simulink model "kalman"  (R2026a)
settings: Solver=FixedStepAuto  StopTime=inf  FixedStep=0.01  EnableMultiTasking=on
libraries: stm32f4xxblockslib x1, stm32blockslib x1
settings Model: STM32="{\"AnalogInput\":{\"ID\":\"1\"},\"TimerCapture\":{\"ID\":\"18\"}}"  SimulationMode=external  Creator=khunb  LastModifiedBy=POND
settings OptimizationCC: MaxStackSize=512
settings HardwareCC: ProdLargestAtomicInteger=Long  ProdLargestAtomicFloat=Double  ProdHWDeviceType=ARM Compatible->ARM Cortex-M
settings SFSimCC: SimCustomHeaderCode="#include \"hc_sr04.h\""  SimUserSources=hc_sr04.c
settings RTWCC: SystemTargetFile=ert.tlc  HardwareBoard=STM32G4xx Based  TLCOptions=-aInlineSetEventsForThisBaseRateFcn=TLC_FALSE -aSuppressMultiTaskScheduler=TLC_FALSE -aRateBasedStepFcn=1  RTWUseSimCustomCode=on  CustomHeaderCode="#include \"hc_sr04.h\""  CustomSource=hc_sr04.c  Toolchain=GNU Tools for STM32  Description=Embedded Coder
settings ERTTargetCC: ExtModeTransport=3.0  ExtModeStaticAllocSize=2048.0  CodeReplacementLibrary=ARM Cortex-M

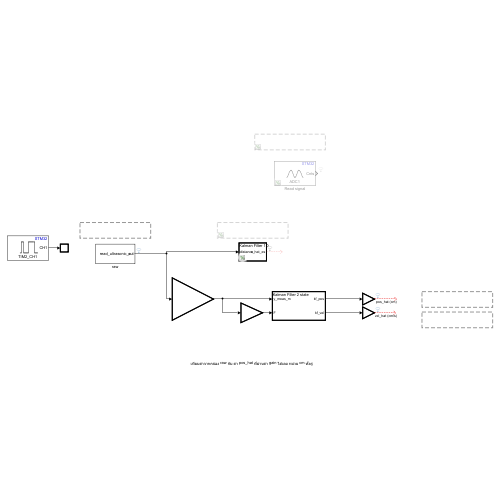
[thumbnail: Simulink's stored preview of the top-level diagram]
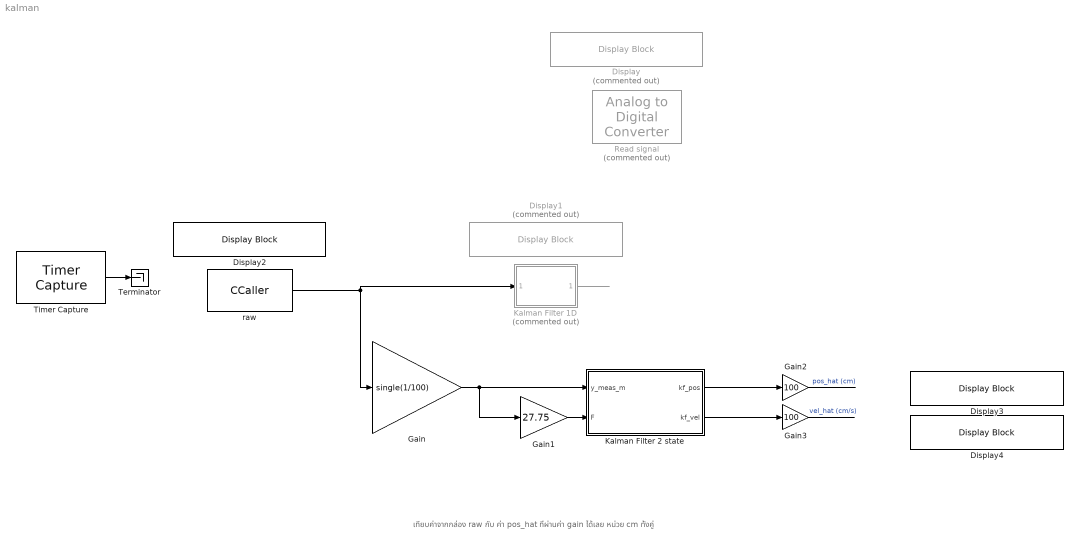
== system kalman ==
  note: เทียบค่าจากกล่อง raw กับ ค่า pos_hat ที่ผ่านค่า gain ได้เลย หน่วย cm ทั้งคู่
  Display : DisplayBlock  Commented=on  LabelPosition=Hide  Transparency=1  GridColor=[0.502, 0.502, 0.502]
  Display1 : DisplayBlock  Commented=on  LabelPosition=Hide  Transparency=1  GridColor=[0.502, 0.502, 0.502]
  Display2 : DisplayBlock  LabelPosition=Hide  Transparency=1  GridColor=[0.502, 0.502, 0.502]
  Display3 : DisplayBlock  LabelPosition=Hide  Transparency=1  GridColor=[0.502, 0.502, 0.502]
  Display4 : DisplayBlock  LabelPosition=Hide  Transparency=1  GridColor=[0.502, 0.502, 0.502]
  Gain : Gain  Gain=single(1/100)
  Gain1 : Gain  Gain=27.75
  Gain2 : Gain  Gain=100
  Gain3 : Gain  Gain=100
  Kalman Filter 1D : MATLAB Function  Commented=on  TreatAsAtomicUnit=on
  Kalman Filter 2 state : MATLAB Function  TreatAsAtomicUnit=on
  Read signal : stm32f4xxblockslib/Analog to Digital Converter  Commented=on  ADCModule=ADC1  ConversionGroup=Regular  TriggerMode=Trigger and read  NumberOfConversions=1  EnableBufferConv=off  BufferLength=1  OutputStatus=off  SampleTime=-1  EnableSimPort=off  hoistedMaskSrc=ECSoC/ECSimCodegen/Analog to Digital Converter
  Terminator : Terminator
  Timer Capture : stm32blockslib/Timer Capture  TimerModule=TIM2  SelectedChannel=CH1  CaptureLength=1  OutputDataLength=off  OutputOverrunStatus=off  OutputDirection=off  SampleTime=-1
      settings: LibrarySourceBlock=stm32g4xxblockslib/Timer Capture
  raw : CCaller  FunctionName=read_ultrasonic_c  PortSpecificationStruct="%)30     .    & (   8    (     @         %    \"     $    !     0         %  0 \"0    $    _    07)G3F%M90  4&]R=$YA;64 4V-O<&4     26YD97@     5'EP90      4VEZ90      27-';&]B86P   X    P    !@    @    $          4    (     0    ,    !         !   P!O=70 #@   #     &    \"     0         !0    @    !     P    $         $  # &]U=  .    .     8    (    !          %    \"     $    &     0         0    !@   $]U='!U=   #@   #@    &    \"     8         !0    @    !     0    $         \"0    @               X    X    !@    @    $          4    (     0    8    !         !     &    <VEN9VQE   .    ,     8    (    !          %    \"     $    !     0         0  $ ,0    X    P    !@    @    ) @        4    (     0    $    !          (  0"
  wires:
  Kalman Filter 1D/1(x_hat_es) -> ?
  raw/1 -> Kalman Filter 1D/1(distance), Gain/1
  Timer Capture/1 -> Terminator/1
  Kalman Filter 2 state/1(kf_pos) -> Gain2/1
  Kalman Filter 2 state/2(kf_vel) -> Gain3/1
  Gain/1 -> Kalman Filter 2 state/1(y_meas_m), Gain1/1
  Gain1/1 -> Kalman Filter 2 state/2(F)
  Gain2/1 -> ?  "pos_hat (cm)"
  Gain3/1 -> ?  "vel_hat (cm/s)"

== matlab function kalman/Kalman Filter 1D ==
  data: distance input; x_hat_es output
function x_hat_es = fcn(distance)
z = double(distance);
Q = 0; % noise covarient
R = 0.0015; % measurement covarient
persistent x_hat P
if isempty(x_hat)
    x_hat = 5; %ค่า estimate เริ่มต้นปรับเอาเลย เดาเลขขึ้นมาได้เลย
    P = 0.0125;% estimate measurement covarient
end
P = P + Q;
K = P / (P+R);
x_hat = x_hat + K * (z - x_hat);
P = (1- K) * P;
x_hat_es =x_hat;

== matlab function kalman/Kalman Filter 2 state ==
  data: y_meas_m input; kf_pos output; F input; kf_vel output
function [kf_pos, kf_vel] = stm32_kalman(y_meas_m, F)
    % --- Physical Parameters (ตรงกับบอร์ด) ---
    m = (150 + 38*5) / 1000;
    k = 27.7465;
    b = 0.082;
    Ts = 0.01;
    y_meas_m  = double(y_meas_m);
    F = double(F);
    % --- ประกาศตัวแปรเก็บสถานะ (เทียบเท่า Global variable ใน C) ---
    persistent x_hat P Q R A B C

    % --- Initialization (ทำงานแค่ครั้งแรก Loop เดียว) ---
    if isempty(x_hat)
        % Initial State & Covariance
        x_hat = [0; 0];
        P = [1 0;
             0 1];
        
        % Noise Matrices (อ้างอิงจาก kalman.c ล่าสุดของคุณ)
        Q = [1e-5, 0; 
             0,   1e-4];
        R = 1.1482157e-04;
        
        % C Matrix (วัดแค่ตำแหน่ง)
        C = [1, 0];
        
        % Discretize A and B Matrices (Euler Forward เหมือนในโค้ด C)
        A = [1,               Ts; 
             -(k/m)*Ts, 1 - (b/m)*Ts];
             
        B = [0; 
             (1/m)*Ts];
    end

    % --- 1. PREDICT ---
    x_pred = A * x_hat + B * F;
    P_pred = A * P * A' + Q;

    % --- 2. KALMAN GAIN ---
    S = C * P_pred * C' + R;
    K = P_pred * C' / S;

    % --- 3. UPDATE ---
    innov = y_meas_m - (C * x_pred);
    x_hat = x_pred + K * innov;
    
    % อัปเดต P matrix: P = (I - K*C)*P_pred
    P = (eye(2) - K * C) * P_pred;

    % --- OUTPUT ---
    kf_pos = x_hat(1);
    kf_vel = x_hat(2);
end
